simulink model "mech_dpend_forw"  (Simulink 6.0)
settings: Solver=ode45  StartTime=0.0  StopTime=10.0  RelTol=1e-3  AbsTol=1e-3
libraries: mblibv1 x6
settings Model: Creator=paulk  LastModifiedBy=batserve  ExtModeAutoUpdateStatusClock=off  BufferReuse=off
settings DataIOCC: SignalLoggingName=sigsOut
settings OptimizationCC: BooleanDataType=off  OptimizeBlockIOStorage=off  BufferReuse=off  ExpressionFolding=off  LocalBlockOutputs=off
settings DebuggingCC: CheckExecutionContextPreStartOutputMsg=on  CheckExecutionContextRuntimeOutputMsg=on  SolverPrmCheckMsg=none
settings HardwareCC: TargetUnknown=on
settings SimMechanicsCC: VisOnUpdateDiagram=on  VisDuringSimulation=on

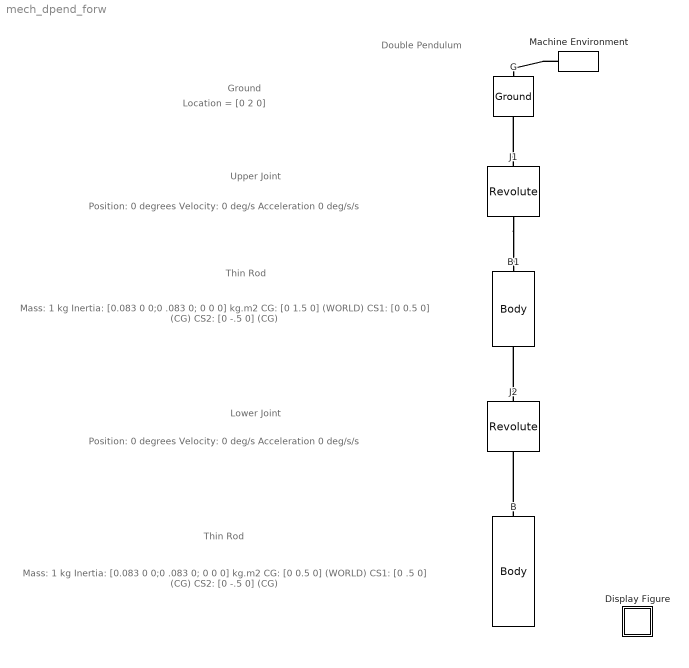
== system mech_dpend_forw ==
  note: Location = [0 2 0]
  note: Mass: 1 kg
      | Inertia: [0.083 0 0;0 .083  0; 0 0 0] kg.m2
      | CG: [0 1.5 0] (WORLD)
      | CS1: [0 0.5 0] (CG)
      | CS2: [0 -.5 0] (CG)
  note: Mass: 1 kg
      | Inertia: [0.083 0 0;0 .083  0; 0 0 0] kg.m2
      | CG: [0 0.5 0] (WORLD)
      | CS1: [0 .5 0] (CG)
      | CS2: [0 -.5 0] (CG)
  note: Position: 0 degrees
      | Velocity: 0 deg/s
      | Acceleration 0 deg/s/s
  note: Position: 0 degrees
      | Velocity: 0 deg/s
      | Acceleration 0 deg/s/s
  note: Ground
  note: Upper Joint
  note: Thin Rod
  note: Thin Rod
  note: Lower Joint
  note: Double Pendulum
  B : mblibv1/Bodies/Body  Orientation=down  PhysicalDomain=mechanical  SubClassName=Unknown  LeftPortType=workingframe  RightPortType=workingframe  LConnTagsString=CS1  DialogClass=MechanicalBodyBlock  Mass=1  MassUnits=kg  InertiaUnits=kg*m^2  Inertia="[0.083 0 0;0 .083  0; 0 0 0]"  Shape=Cylinder  ShapeDims=[1 1]  ShapeUnits=m  ShapeUse=false  Density=1  DensityUnits=kg/m^3  DensityUse=false  CG=Left$CG$[0 .5 0]$WORLD$WORLD$m$[0 0 0]$Euler X-Y-Z$deg$WORLD$false  WorkingFrames=Left$CS1$[0 .5 0]$CG$CG$m$[0 0 0]$Euler X-Y-Z$deg$WORLD$true#Right$CS2$[0 -.5 0]$CG$CG$m$[0 0 0]$Euler X-Y-Z$deg$WORLD$false
  B1 : mblibv1/Bodies/Body  Orientation=down  PhysicalDomain=mechanical  SubClassName=Unknown  LeftPortType=workingframe  RightPortType=workingframe  LConnTagsString=CS1  RConnTagsString=CS2  DialogClass=MechanicalBodyBlock  Mass=1  MassUnits=kg  InertiaUnits=kg*m^2  Inertia="[0.083 0 0;0 .083  0; 0 0 0]"  Shape=Cylinder  ShapeDims=[1 1]  ShapeUnits=m  ShapeUse=false  Density=1  DensityUnits=kg/m^3  DensityUse=false  CG=Left$CG$[0 1.5 0]$WORLD$WORLD$m$[0 0 0]$Euler X-Y-Z$deg$WORLD$false  WorkingFrames=Left$CS1$[0 .5 0]$CG$CG$m$[0 0 0]$Euler X-Y-Z$deg$WORLD$true#Right$CS2$[0 -.5 0]$CG$CG$m$[0 0 0]$Euler X-Y-Z$deg$WORLD$true
  Display Figure : Subsystem  Tag=Help  Description="Help callback for forward dynamics double pendulum model: mech_dpend_forw.  Opens Help browser to Type 19 marker at documentation for this tutorial model."
      settings: OpenFcn=pmhelpview([docroot '/toolbox/physmod/mech/mech.map'], 'mech_dpend_forw_help');
      mask Type: Help callback
      mask Display: image(imread('info.bmp'))
  G : mblibv1/Bodies/Ground  Orientation=down  Opaque=on  LeftPortType=env  RightPortType=workingframe  PhysicalDomain=Mechanical  DialogClass=GroundBlock  CoordPosition=[0 2 0]  CoordPositionUnits=m  StateVectorMgrId=-1  MachineId=[0 0]  ShowEnvPort=on
  J1 : mblibv1/Joints/Revolute  Orientation=down  PhysicalDomain=mechanical  SubClassName=Unknown  LeftPortType=blob  RightPortType=blob  LConnTagsString=__newl0  RConnTagsString=__newr0  NumSAPorts=0  CutJoint=off  MarkAsCut=off  Primitives=revolute  PrimitiveProps=R1$WORLD$[0 0 1]$revolute  DialogClass=JointBlock
  J2 : mblibv1/Joints/Revolute  Orientation=down  PhysicalDomain=mechanical  SubClassName=Unknown  LeftPortType=blob  RightPortType=blob  LConnTagsString=__newl0  RConnTagsString=__newr0  NumSAPorts=0  CutJoint=off  MarkAsCut=off  Primitives=revolute  PrimitiveProps=R1$WORLD$[0 0 1]$revolute  DialogClass=JointBlock
  Machine Environment : mblibv1/Bodies/Machine Environment  Tag=Factory ground  Orientation=left  DialogController=MECH.DialogSource  Opaque=on  PortType=env  PhysicalDomain=Mechanical  DialogTemplateClass=MECH.MachineEnvironment  SyncWhenCopied=off  Gravity=[0 -9.81 0]  GravityUnits=m/s^2  GravityAsSignal=off  Dimensionality=3D Only  AnalysisType=Forward dynamics  LinearAssemblyTolerance=1e-3  LinearAssemblyToleranceUnits=m  AngularAssemblyTolerance=1e-3  AngularAssemblyToleranceUnits=rad  ConstraintSolverType=Stabilizing  ConstraintRelTolerance=1e-4  ConstraintAbsTolerance=1e-4  UseRobustSingularityHandling=off  StatePerturbationType=Fixed  PerturbationSize=1e-5  VisualizeMachine=on
  connections:
  J1/LConn1 -- G/RConn1
  J1/RConn1 -- B1/LConn1
  B/LConn1 -- J2/RConn1
  J2/LConn1 -- B1/RConn1
  Machine Environment/RConn1 -- G/LConn1

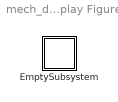
== system mech_dpend_forw/Display Figure ==
  EmptySubsystem : Subsystem

== system mech_dpend_forw/Display Figure/EmptySubsystem ==
